simulink model "bloques"  (R2022a)
settings: Solver=VariableStepAuto  StartTime=0.0  StopTime=150  RelTol=1e-3
settings Model: Creator=angel  LastModifiedBy=angel

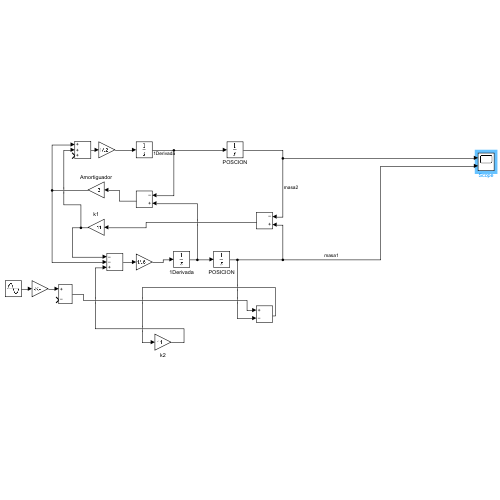
[thumbnail: Simulink's stored preview of the top-level diagram]
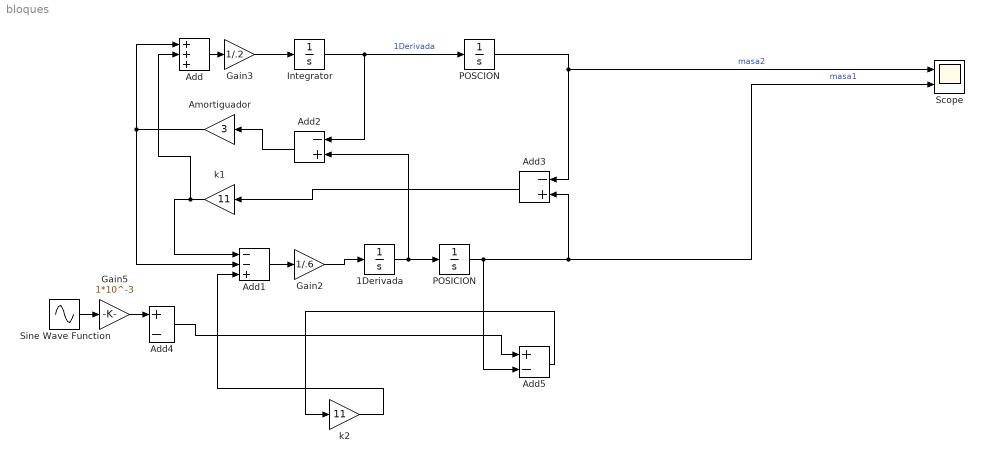
== system bloques ==
  1Derivada : Integrator
  Add : Sum  Inputs=+++
  Add1 : Sum  Inputs=--+
  Add2 : Sum  Inputs=-+
  Add3 : Sum  Inputs=-+
  Add4 : Sum  Inputs=+-
  Add5 : Sum  Inputs=+-
  Amortiguador : Gain  Gain=3
  Gain2 : Gain  Gain=1/.6
  Gain3 : Gain  Gain=1/.2
  Gain5 : Gain  Gain=1*10^-3
  Integrator : Integrator
  POSCION : Integrator
  POSICION : Integrator
  Scope : Scope  NumInputPorts=2
  Sine Wave Function : Sin  Amplitude=137  Frequency=.7*pi  SampleTime=0
  k1 : Gain  Gain=11
  k2 : Gain  Gain=11
  wires:
  Add4/1 -> Add5/1
  Integrator/1 -> POSCION/1, Add2/1  "1Derivada"
  POSCION/1 -> Add3/1, Scope/1  "masa2"
  1Derivada/1 -> POSICION/1, Add2/2
  Add1/1 -> Gain2/1
  Add3/1 -> k1/1
  Add2/1 -> Amortiguador/1
  Amortiguador/1 -> Add1/2, Add/1
  Gain2/1 -> 1Derivada/1
  Gain3/1 -> Integrator/1
  Add/1 -> Gain3/1
  Add5/1 -> k2/1
  k2/1 -> Add1/3
  POSICION/1 -> Scope/2, Add3/2, Add5/2  "masa1"
  k1/1 -> Add/2, Add1/1
  Sine Wave Function/1 -> Gain5/1
  Gain5/1 -> Add4/1
